simulink model "one_axis_servo_i_ff"  (R2024b)
settings: Solver=VariableStepAuto  StartTime=0.0  StopTime=10.0  RelTol=1e-3
values from neighbouring files (symbols this model uses):
  Kpp = 40    [check_2dof_model.m]    (also in ex8_4.m = 4; ex9.m; load_ex9_model.m)
  Kvf = 0.7    [check_2dof_model.m]    (also in ex9.m; load_ex9_model.m)
settings Model: Creator=shohei  LastModifiedBy=shohei

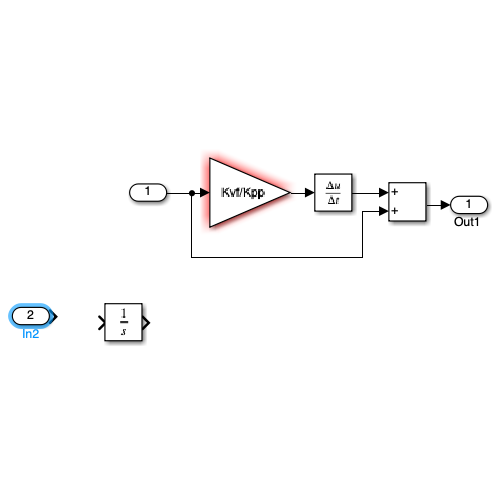
[thumbnail: Simulink's stored preview of the top-level diagram]
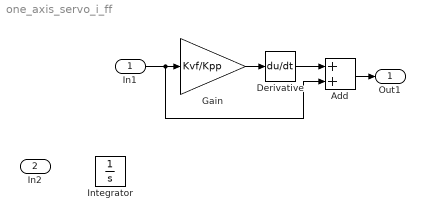
== system one_axis_servo_i_ff ==
  In1 : Inport
  In2 : Inport  Port=2
  Add : Sum
  Derivative : Derivative
  Gain : Gain  Gain=Kvf/Kpp
  Integrator : Integrator
  "Out1 " : Outport
  wires:
  Gain/1 -> Derivative/1
  Derivative/1 -> Add/1
  Add/1 -> "Out1 "/1
  In1/1 -> Add/2, Gain/1
